simulink model "Model_mnogocanal_system_svyazi_s_vrem_razd_canalov"  (R2023b)
settings: Solver=VariableStepAuto  StartTime=0.0  StopTime=0.000005  RelTol=1e-3
libraries: dspfdesign x6, simulink x2
settings Model: Creator=User  LastModifiedBy=User

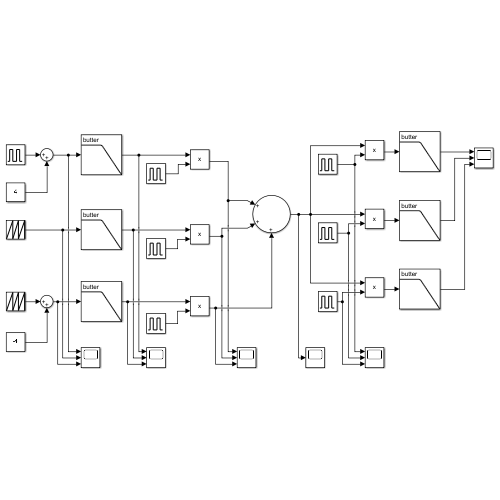
[thumbnail: Simulink's stored preview of the top-level diagram]
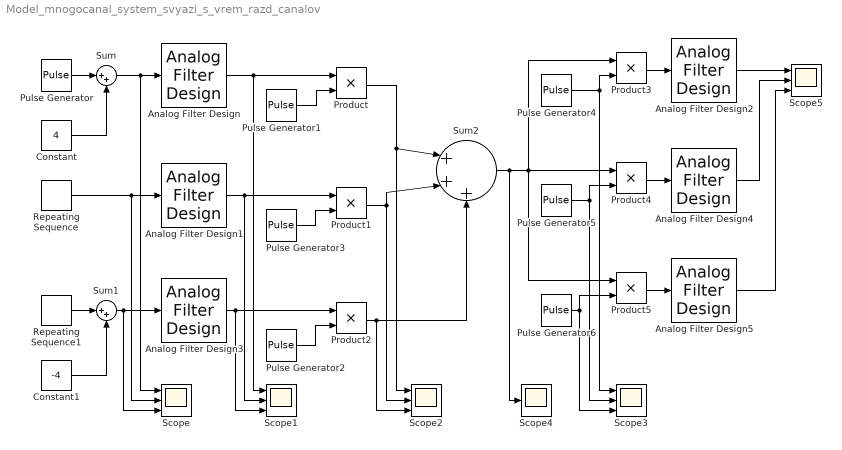
== system Model_mnogocanal_system_svyazi_s_vrem_razd_canalov ==
  Analog Filter Design{,1..5} (6 alike) : dspfdesign/Analog Filter Design  method=Butterworth  filttype=Lowpass  N=8  Wlo=30  Whi=80  Rp=2  Rs=40
  Constant : Constant  Value=4
  Constant1 : Constant  Value=-4
  Product{,1..5} (6 alike) : Product
  Pulse Generator{,1..6} (7 alike) : DiscretePulseGenerator  PulseType=Time based  Amplitude=3  Period=0.4*10^(-6)  PulseWidth=50
  Repeating Sequence : simulink/Sources/Repeating Sequence  rep_seq_t=[0 2*10^(-6)]  rep_seq_y=[0 3]
  Repeating Sequence1 : simulink/Sources/Repeating Sequence  rep_seq_t=[0 0.3*10^(-6)]  rep_seq_y=[0 4.5]
  Scope{,1..3,5} (5 alike) : Scope  NumInputPorts=3
  Scope4 : Scope
  Sum : Sum  Inputs=|++
  Sum1 : Sum  Inputs=|++
  Sum2 : Sum  Inputs=|+++
  wires:
  Pulse Generator/1 -> Sum/1
  Constant/1 -> Sum/2
  Repeating Sequence/1 -> Analog Filter Design1/1, Scope/2
  Sum/1 -> Analog Filter Design/1, Scope/1
  Repeating Sequence1/1 -> Sum1/1
  Constant1/1 -> Sum1/2
  Sum1/1 -> Analog Filter Design3/1, Scope/3
  Analog Filter Design2/1 -> Scope5/1
  Analog Filter Design4/1 -> Scope5/2
  Analog Filter Design5/1 -> Scope5/3
  Product5/1 -> Analog Filter Design5/1
  Product3/1 -> Analog Filter Design2/1
  Product4/1 -> Analog Filter Design4/1
  Pulse Generator5/1 -> Product4/2, Scope3/2
  Pulse Generator4/1 -> Product3/2, Scope3/1
  Pulse Generator6/1 -> Product5/2, Scope3/3
  Sum2/1 -> Scope4/1, Product4/1, Product3/1, Product5/1
  Pulse Generator3/1 -> Product1/2
  Pulse Generator2/1 -> Product2/2
  Pulse Generator1/1 -> Product/2
  Analog Filter Design3/1 -> Product2/1, Scope1/3
  Analog Filter Design1/1 -> Product1/1, Scope1/2
  Analog Filter Design/1 -> Product/1, Scope1/1
  Product2/1 -> Sum2/3, Scope2/3
  Product1/1 -> Scope2/2, Sum2/2
  Product/1 -> Scope2/1, Sum2/1
